simulink model "GroundControl"  (R2020b)
settings: Solver=VariableStepAuto  StartTime=0.0  StopTime=10.0  RelTol=1e-3
libraries: uavmavlinklib x2
settings Model: Creator=macra  LastModifiedBy=macra

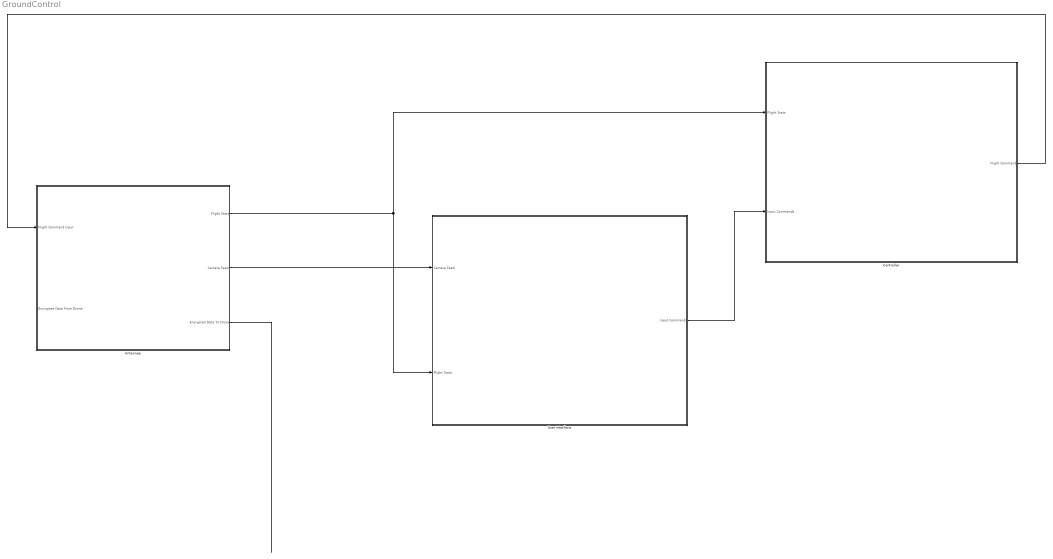
== system GroundControl ==
  Antennae : Subsystem
  Controller : Subsystem
  User Interface : Subsystem
  wires:
  Antennae/1(Flight Stats) -> User Interface/2(Flight Stats), Controller/1(Flight Stats)
  Antennae/2(Camera Feed) -> User Interface/1(Camera Feed)
  User Interface/1(Input Commands) -> Controller/2(Input Commands)
  Controller/1(Flight Command) -> Antennae/1(Flight Command Input)
  Antennae/3("Encrypted Data To Drone ") -> ?
  ? -> Antennae/2(Encrypted Data From Drone)

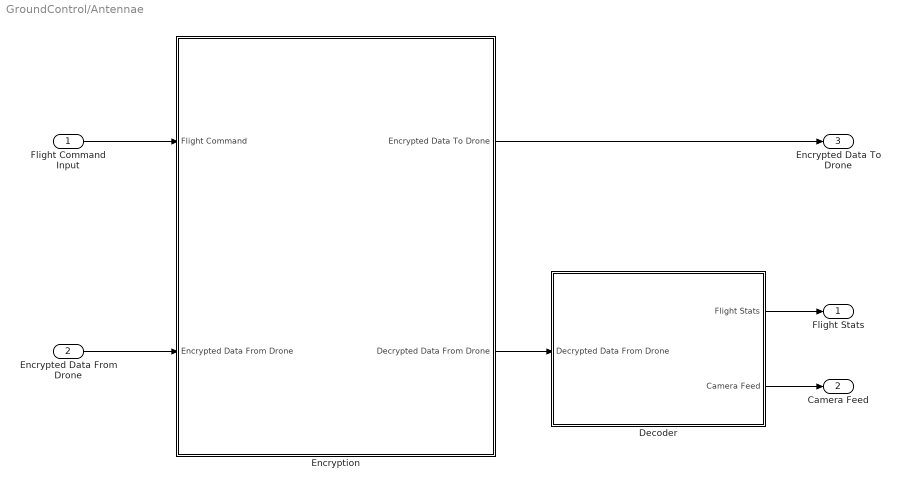
== system GroundControl/Antennae ==
  Flight Command Input : Inport
  Encrypted Data From Drone : Inport  Port=2
  Decoder : Subsystem
  Encryption : Subsystem
  Flight Stats : Outport
  Camera Feed : Outport  Port=2
  "Encrypted Data To Drone " : Outport  Port=3
  wires:
  Flight Command Input/1 -> Encryption/1(Flight Command)
  Encrypted Data From Drone/1 -> Encryption/2(Encrypted Data From Drone)
  Encryption/2(Decrypted Data From Drone) -> Decoder/1(Decrypted Data From Drone)
  Decoder/1(Flight Stats) -> Flight Stats/1
  Decoder/2(Camera Feed) -> Camera Feed/1
  Encryption/1("Encrypted Data To Drone ") -> "Encrypted Data To Drone "/1

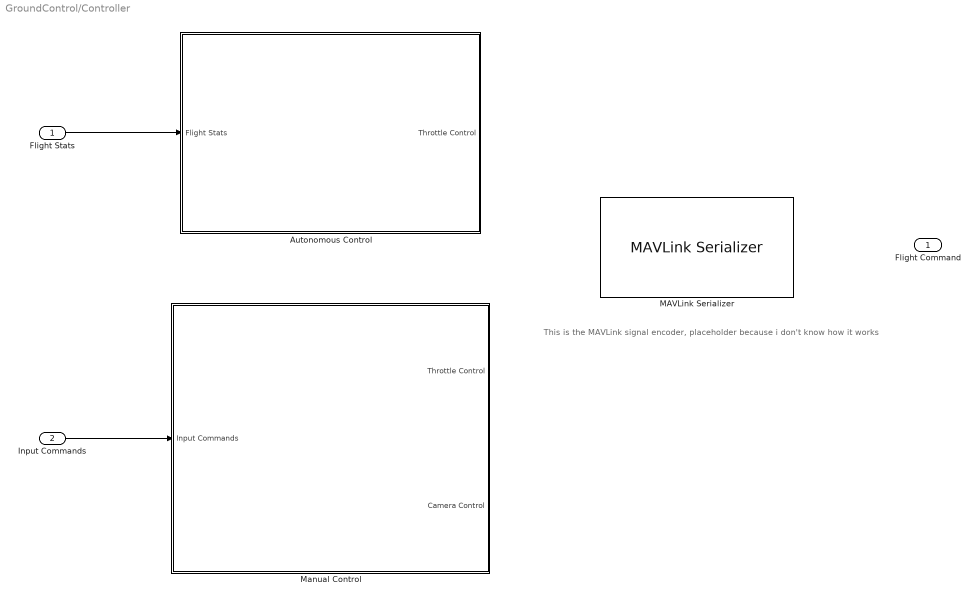
== system GroundControl/Controller ==
  note: This is the MAVLink signal encoder, placeholder
      | because i don't know how it works
  Flight Stats : Inport
  Input Commands : Inport  Port=2
  Autonomous Control : Subsystem
  MAVLink Serializer : uavmavlinklib/MAVLink Serializer  dialectSource=Select from standard MAVLink dialects  dialect=common.xml  dialectCustom=common.xml  version=2  messageType=HEARTBEAT
      settings: SourceProductBaseCode=UV
  Manual Control : Subsystem
  Flight Command : Outport
  wires:
  Input Commands/1 -> Manual Control/1(Input Commands)
  Flight Stats/1 -> Autonomous Control/1(Flight Stats)

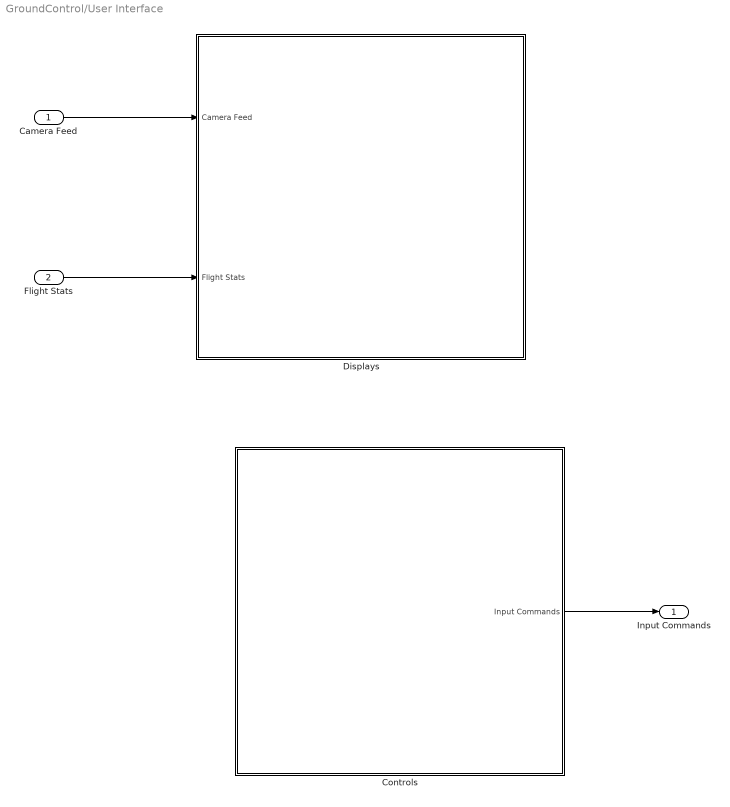
== system GroundControl/User Interface ==
  Camera Feed : Inport
  Flight Stats : Inport  Port=2
  Controls : Subsystem
  Displays : Subsystem
  Input Commands : Outport
  wires:
  Camera Feed/1 -> Displays/1(Camera Feed)
  Flight Stats/1 -> Displays/2(Flight Stats)
  Controls/1(Input Commands) -> Input Commands/1

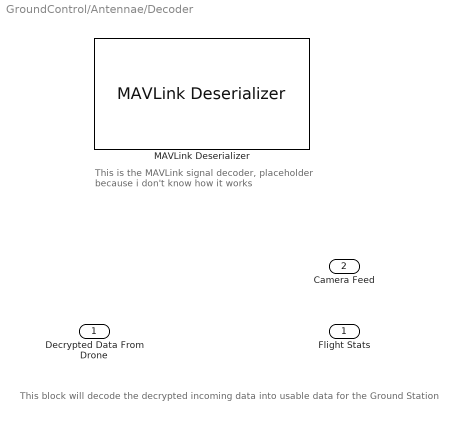
== system GroundControl/Antennae/Decoder ==
  note: This is the MAVLink signal decoder, placeholder
      | because i don't know how it works
  note: This block will decode the decrypted incoming data into usable data for the Ground Station
  Decrypted Data From Drone : Inport
  MAVLink Deserializer : uavmavlinklib/MAVLink Deserializer  dialectSource=Select from standard MAVLink dialects  dialect=common.xml  dialectCustom=common.xml  version=2  messageType=HEARTBEAT  inputDataLength=off  SystemIDFilter=off  systemID=1  ComponentIDFilter=off  componentID=1  queueMsg=off  queueMsgSize=50  dropNum=off
      settings: SourceProductBaseCode=UV
  Flight Stats : Outport
  Camera Feed : Outport  Port=2

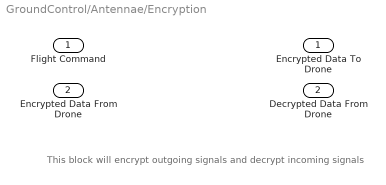
== system GroundControl/Antennae/Encryption ==
  note: This block will encrypt outgoing signals and decrypt incoming signals
  Flight Command : Inport
  Encrypted Data From Drone : Inport  Port=2
  "Encrypted Data To Drone " : Outport
  Decrypted Data From Drone : Outport  Port=2

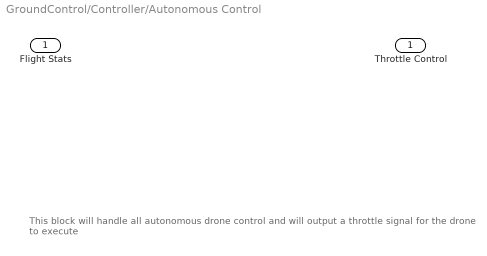
== system GroundControl/Controller/Autonomous Control ==
  note: This block will handle all autonomous drone control and will output a throttle signal for the drone to execute
  Flight Stats : Inport
  Throttle Control : Outport

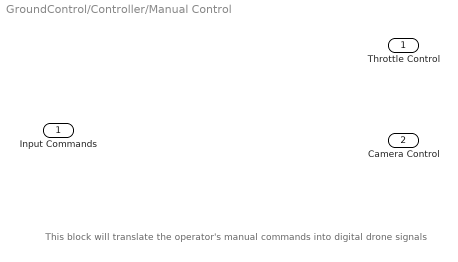
== system GroundControl/Controller/Manual Control ==
  note: This block will translate the operator's manual commands into digital drone signals
  Input Commands : Inport
  Throttle Control : Outport
  Camera Control : Outport  Port=2

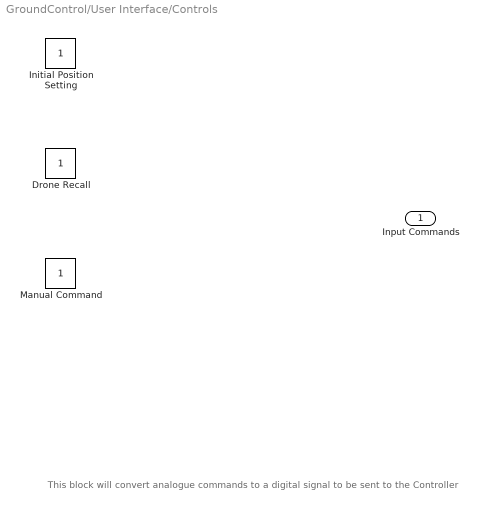
== system GroundControl/User Interface/Controls ==
  note: This block will convert analogue commands to a digital signal to be sent to the Controller
  Drone Recall : Constant
  Initial Position Setting : Constant
  Manual Command : Constant
  Input Commands : Outport

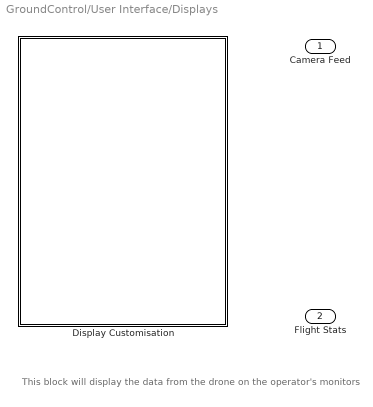
== system GroundControl/User Interface/Displays ==
  note: This block will display the data from the drone on the operator's monitors
  Camera Feed : Inport
  Flight Stats : Inport  Port=2
  Display Customisation : Subsystem

== system GroundControl/User Interface/Displays/Display Customisation ==
  note: This block will allow the display configuration to be customized
